simulink model "CompLab1_2"  (R2020a)
settings: Solver=VariableStepAuto  StartTime=0.0  StopTime=10.0  RelTol=1e-3
undefined symbols (not defined in the file): b, dx0, extforce, k, m, stepi, stept, x0
settings Model: Creator=cal  LastModifiedBy=cal
settings DataIOCC: ReturnWorkspaceOutputs=off  TimeSaveName=mytime

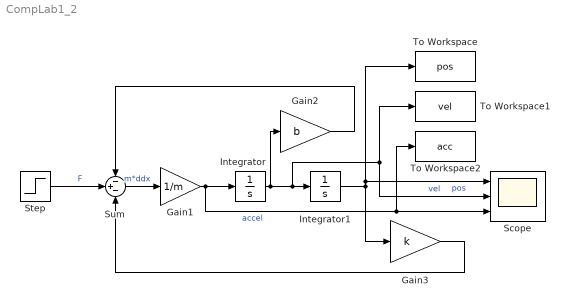
== system CompLab1_2 ==
  Gain1 : Gain  Gain=1/m
  Gain2 : Gain  Gain=b
  Gain3 : Gain  Gain=k
  Integrator : Integrator  InitialCondition=dx0
  Integrator1 : Integrator  InitialCondition=x0
  Scope : Scope  NumInputPorts=3
  Step : Step  Time=stept  Before=stepi  After=extforce  SampleTime=0
  Sum : Sum  Inputs=-+-
  To Workspace : ToWorkspace  VariableName=pos  SampleTime=-1
  To Workspace1 : ToWorkspace  VariableName=vel  SampleTime=-1
  To Workspace2 : ToWorkspace  VariableName=acc  SampleTime=-1
  wires:
  Integrator/1 -> Gain2/1, To Workspace1/1, Scope/2, Integrator1/1  "vel"
  Step/1 -> Sum/2  "F"
  Sum/1 -> Gain1/1  "m*ddx"
  Gain1/1 -> Integrator/1, To Workspace2/1, Scope/3  "accel"
  Integrator1/1 -> Gain3/1, To Workspace/1, Scope/1  "pos"
  Gain2/1 -> Sum/1
  Gain3/1 -> Sum/3
